simulink model "Rlocus"  (R2021a)
settings: Solver=VariableStepAuto  StartTime=0.0  StopTime=10.0  RelTol=1e-3
settings Model: Creator=User  LastModifiedBy=User

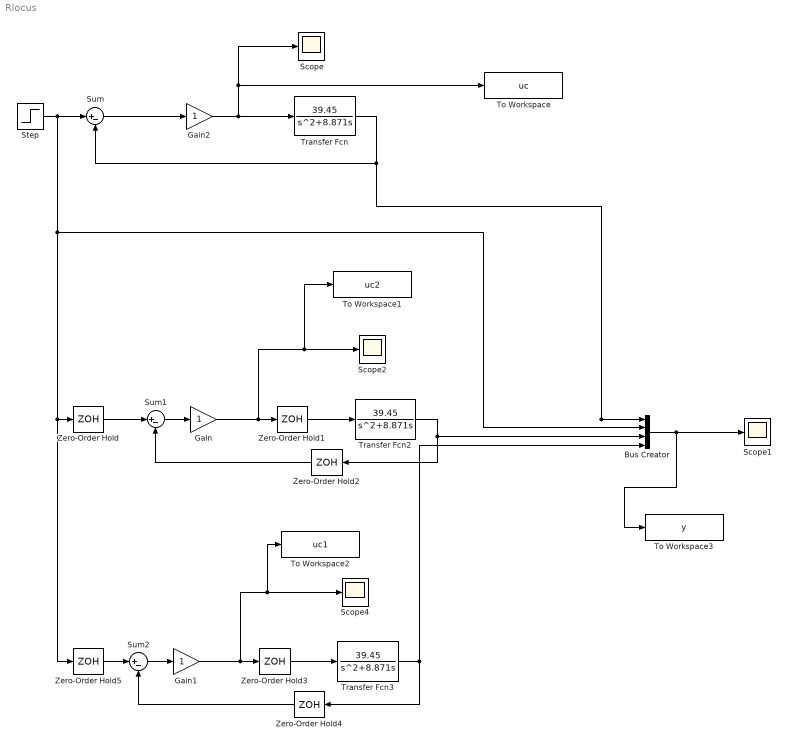
== system Rlocus ==
  Bus Creator : BusCreator  Inputs=4
  Gain : Gain
  Gain1 : Gain
  Gain2 : Gain
  Scope{,1..2,4} (4 alike) : Scope
  Step : Step  SampleTime=0
  Sum : Sum  Inputs=|+-
  Sum1 : Sum  Inputs=|+-
  Sum2 : Sum  Inputs=|+-
  To Workspace : ToWorkspace  VariableName=uc  SaveFormat=Timeseries  SampleTime=-1
  To Workspace1 : ToWorkspace  VariableName=uc2  SaveFormat=Timeseries  SampleTime=-1
  To Workspace2 : ToWorkspace  VariableName=uc1  SaveFormat=Timeseries  SampleTime=-1
  To Workspace3 : ToWorkspace  VariableName=y  SaveFormat=Timeseries  SampleTime=-1
  Transfer Fcn : TransferFcn  Numerator=[39.45]  Denominator=[1 8.871 0]
  Transfer Fcn2 : TransferFcn  Numerator=[39.45]  Denominator=[1 8.871 0]
  Transfer Fcn3 : TransferFcn  Numerator=[39.45]  Denominator=[1 8.871 0]
  Zero-Order Hold : ZeroOrderHold  SampleTime=0.1
  Zero-Order Hold1 : ZeroOrderHold  SampleTime=0.1
  Zero-Order Hold2 : ZeroOrderHold  SampleTime=0.1
  Zero-Order Hold3 : ZeroOrderHold  SampleTime=0.6
  Zero-Order Hold4 : ZeroOrderHold  SampleTime=0.6
  Zero-Order Hold5 : ZeroOrderHold  SampleTime=0.6
  wires:
  Step/1 -> Zero-Order Hold5/1, Zero-Order Hold/1, Bus Creator/2, Sum/1
  Sum/1 -> Gain2/1
  Transfer Fcn/1 -> Bus Creator/1, Sum/2
  Gain2/1 -> Scope/1, To Workspace/1, Transfer Fcn/1
  Transfer Fcn2/1 -> Zero-Order Hold2/1, Bus Creator/3
  Zero-Order Hold2/1 -> Sum1/2
  Gain/1 -> To Workspace1/1, Scope2/1, Zero-Order Hold1/1
  Zero-Order Hold1/1 -> Transfer Fcn2/1
  Zero-Order Hold4/1 -> Sum2/2
  Sum2/1 -> Gain1/1
  Gain1/1 -> To Workspace2/1, Scope4/1, Zero-Order Hold3/1
  Zero-Order Hold3/1 -> Transfer Fcn3/1
  Zero-Order Hold/1 -> Sum1/1
  Transfer Fcn3/1 -> Bus Creator/4, Zero-Order Hold4/1
  Bus Creator/1 -> To Workspace3/1, Scope1/1
  Sum1/1 -> Gain/1
  Zero-Order Hold5/1 -> Sum2/1
